simulink model "q4_simulink"  (R2023b)
settings: Solver=VariableStepAuto  StartTime=0.0  StopTime=5  RelTol=1e-3
values from neighbouring files (symbols this model uses):
  A = [0, 1,      0;       0, -b/J,   K/J;       0, -K/L, -R/L;]    [lec7_dc_motor_control_example.m]    (also in lec7_example_11.m = [0 0 4 1; lec7_notes_example_11.m = [-1, 1, 0;       0,  1, 1;       0,  0, 2;]; mini_proj_1.m = [-8.8487 + (a-b)/5,     -0.0399,              -5.55 + (c+d)/; mini_proj_q1.m = [-8.8487 + (a-b)/5,     -0.0399,              -5.55 + (c+d)/)
  B = [0;       0;       1/L;]    [lec7_dc_motor_control_example.m]    (also in lec7_example_11.m = [-2 0; lec7_notes_example_11.m = [1, 1;       0, 0;       0, 1;]; mini_proj_1.m = [0.0564+(b)/(10+c),           0.0319;       0.0165-(c+d-5)/(; mini_proj_q1.m = [0.0564+(b)/(10+c),           0.0319)
  C = [1, 0, 0]    [lec7_dc_motor_control_example.m]    (also in lec7_notes_example_11.m = [1, 3, -1;      0, 1,  0;]; mini_proj_1.m = [-3.2988,           -2.1932+(10*c+d)/(100+5*a), 0.0370,  -0.; mini_proj_q1.m = [-3.2988,           -2.1932+(10*c+d)/(100+5*a), 0.0370,  -0.; mini_proj_q2.m = [-3.2988,           -2.1932+(10*c+d)/(100+5*a), 0.0370,  -0.)
  F = inv(B_star)    [q4_full.m]
  K = transpose(place(A, B, des_poles))    [lec7_dc_motor_control_example.m]    (also in lec7_example_11.m = K_bar * T; lec7_notes_example_11.m = K_bar * T; mini_proj_1.m = K_bar * T; mini_proj_q1.m = K_bar * T)
  x_0 = [0.5; -0.1; 0.3; -0.8;]    [mini_proj_1.m]    (also in mini_proj_q1.m; mini_proj_q2.m; q1_full.m; q1_params.m)
settings Model: Creator=john  LastModifiedBy=john

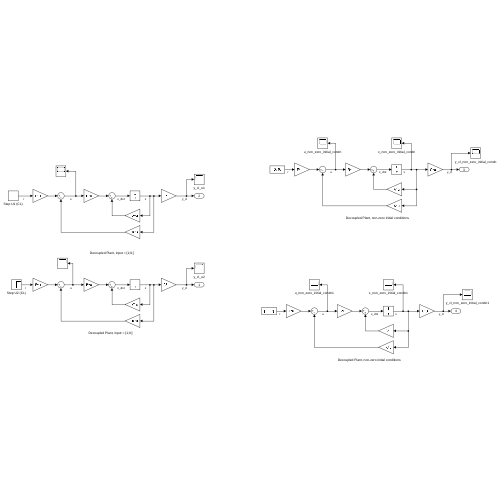
[thumbnail: Simulink's stored preview of the top-level diagram]
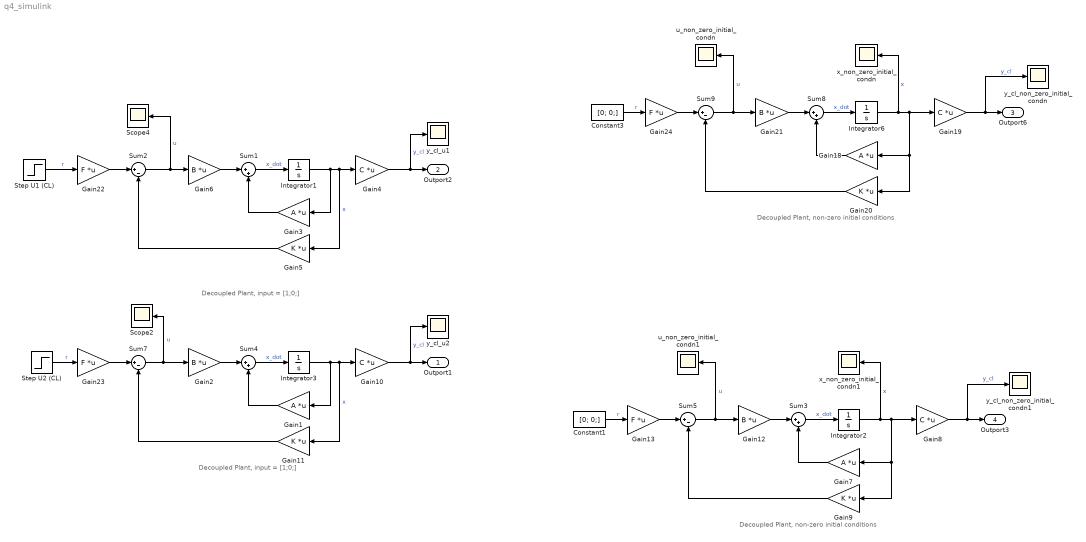
== system q4_simulink ==
  note: Decoupled Plant, input = [1;0;]
  note: Decoupled Plant, input = [1;0;]
  note: Decoupled Plant, non-zero initial conditions
  note: Decoupled Plant, non-zero initial conditions
  Constant1 : Constant  Value=[0; 0;]
  Constant3 : Constant  Value=[0; 0;]
  Gain{1,3,7,18} (4 alike) : Gain  Gain=A  Multiplication=Matrix(K*u)
  Gain{4,8,10,19} (4 alike) : Gain  Gain=C  Multiplication=Matrix(K*u)
  Gain{5,9,11,20} (4 alike) : Gain  Gain=K  Multiplication=Matrix(K*u)
  Gain{2,6,12,21} (4 alike) : Gain  Gain=B  Multiplication=Matrix(K*u)
  Gain{13,22..24} (4 alike) : Gain  Gain=F  Multiplication=Matrix(K*u)
  Integrator1 : Integrator
  Integrator2 : Integrator
  Integrator3 : Integrator
  Integrator6 : Integrator  InitialCondition=x_0
  Scope2 : Scope
  Scope4 : Scope
  Step U1 (CL) : Step  Time=0  Before=[0; 0;];  After=[1; 0;];  SampleTime=0
  Step U2 (CL) : Step  Time=0  Before=[0; 0;];  After=[0; 1;];  SampleTime=0
  Sum{1,3..4,8} (4 alike) : Sum  Inputs=|++
  Sum{2,5,7,9} (4 alike) : Sum  Inputs=|+-
  u_non_zero_initial_condn : Scope
  u_non_zero_initial_condn1 : Scope
  x_non_zero_initial_condn : Scope
  x_non_zero_initial_condn1 : Scope
  y_cl_non_zero_initial_condn : Scope
  y_cl_non_zero_initial_condn1 : Scope
  y_cl_u1 : Scope
  y_cl_u2 : Scope
  Outport1 : Outport
  Outport2 : Outport  Port=2
  Outport6 : Outport  Port=3
  Outport3 : Outport  Port=4
  wires:
  Gain10/1 -> y_cl_u2/1, Outport1/1  "y_cl"
  Integrator3/1 -> Gain1/1, Gain11/1, Gain10/1  "x"
  Gain1/1 -> Sum4/2
  Gain11/1 -> Sum7/2
  Sum4/1 -> Integrator3/1  "x_dot"
  Sum7/1 -> Scope2/1, Gain2/1  "u"
  Step U2 (CL)/1 -> Gain23/1  "r"
  Gain2/1 -> Sum4/1
  Gain4/1 -> y_cl_u1/1, Outport2/1  "y_cl"
  Gain6/1 -> Sum1/1
  Sum1/1 -> Integrator1/1  "x_dot"
  Integrator1/1 -> Gain3/1, Gain5/1, Gain4/1  "x"
  Gain5/1 -> Sum2/2
  Sum2/1 -> Scope4/1, Gain6/1  "u"
  Step U1 (CL)/1 -> Gain22/1  "r"
  Gain3/1 -> Sum1/2
  Gain21/1 -> Sum8/1
  Gain20/1 -> Sum9/2
  Sum8/1 -> Integrator6/1  "x_dot"
  Integrator6/1 -> Gain20/1, Gain18/1, Gain19/1, x_non_zero_initial_condn/1  "x"
  Gain19/1 -> y_cl_non_zero_initial_condn/1, Outport6/1  "y_cl"
  Sum9/1 -> u_non_zero_initial_condn/1, Gain21/1  "u"
  Gain18/1 -> Sum8/2
  Constant3/1 -> Gain24/1  "r"
  Gain22/1 -> Sum2/1
  Gain23/1 -> Sum7/1
  Gain24/1 -> Sum9/1
  Gain8/1 -> y_cl_non_zero_initial_condn1/1, Outport3/1  "y_cl"
  Sum3/1 -> Integrator2/1  "x_dot"
  Gain13/1 -> Sum5/1
  Gain9/1 -> Sum5/2
  Gain7/1 -> Sum3/2
  Constant1/1 -> Gain13/1  "r"
  Gain12/1 -> Sum3/1
  Sum5/1 -> u_non_zero_initial_condn1/1, Gain12/1  "u"
  Integrator2/1 -> Gain9/1, Gain7/1, Gain8/1, x_non_zero_initial_condn1/1  "x"
